simulink model "VFD.Simulink"  (R2022b)
settings: Solver=VariableStepAuto  StartTime=0.0  StopTime=5  RelTol=1e-3
libraries: spsMosfetLib x6, simulink x2, spsAsynchronousMachineSIUnitsLib x1, spsDCVoltageSourceLib x1, sps_lib x1
settings Model: Creator=Raghavendra Margam  LastModifiedBy=Raghavendra Margam

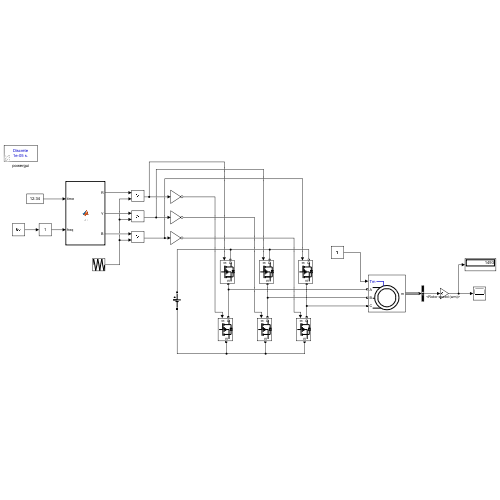
[thumbnail: Simulink's stored preview of the top-level diagram]
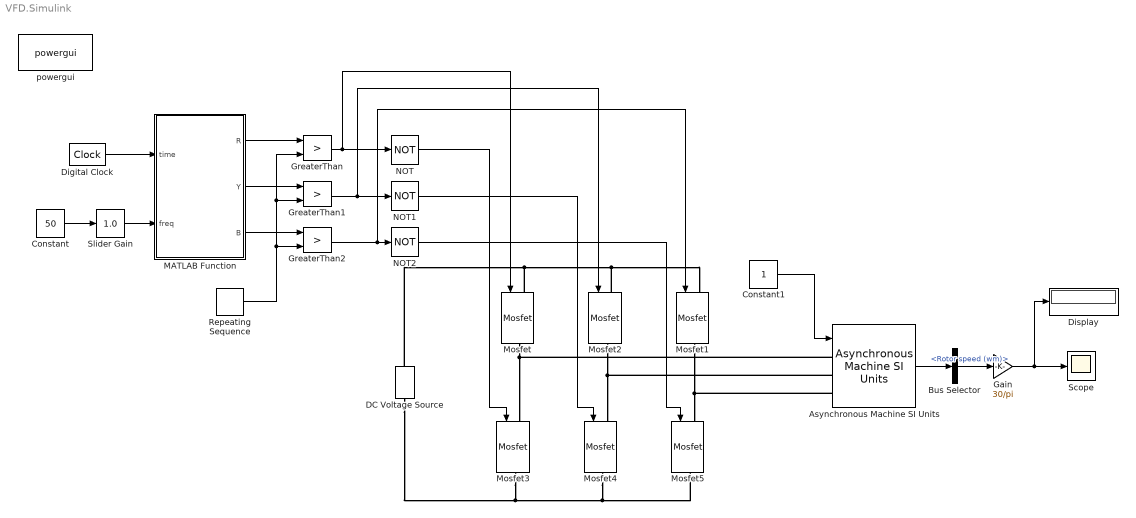
== system VFD.Simulink ==
  Asynchronous Machine SI Units : spsAsynchronousMachineSIUnitsLib/Asynchronous Machine SI Units  RotorType=Squirrel-cage  PresetModel="15:  5.4 HP (4KW)   400 V  50Hz 1430 RPM"  MechanicalLoad=Torque Tm  ShowDetailedParameters=on  ReferenceFrame=Stationary  Units=SI  MeasurementBus=off  NominalParameters=[4000 400 50]  VoltageRatio=1  Stator=[1.405 0.005839]  Rotor=[1.395 0.005839]  Cage1=[-3.163 0.003621]  Cage2=[-18.98 0.001646]  Lm=0.1722  Mechanical=[0.0131 0.002985 2]  PolePairs=2  InitialConditions=[1 0 0 0 0 0 0 0]  SimulateSaturation=off  Saturation=[14.03593122, 27.81365428, 53.79336849, 72.68890987, 97.98006896, 148.6815601, 215.7428561, 302.9841135, 428.7778367 ; 230, 322, 414, 460, 506, 552, 598, 644, 690]  LoadFlowParameters=1492000  TsPowergui=0  TsBlock=-1  IterativeModel=Trapezoidal non iterative  IterativeDiscreteModel=Trapezoidal non iterative  Pmec=1.492e+006
  Bus Selector : BusSelector  OutputSignals=Mechanical.Rotor speed (wm)
  Constant : Constant  Value=50
  Constant1 : Constant
  DC Voltage Source : spsDCVoltageSourceLib/DC Voltage Source  Amplitude=500  Measurements=None
  Digital Clock : DigitalClock  SampleTime=1e-5
  Display : Display
  Gain : Gain  Gain=30/pi
  GreaterThan : RelationalOperator  Operator=>  OutDataTypeStr=boolean  RndMeth=Simplest  InputSameDT=off
  GreaterThan1 : RelationalOperator  Operator=>  OutDataTypeStr=boolean  RndMeth=Simplest  InputSameDT=off
  GreaterThan2 : RelationalOperator  Operator=>  OutDataTypeStr=boolean  RndMeth=Simplest  InputSameDT=off
  MATLAB Function : MATLAB Function  TreatAsAtomicUnit=on
  Mosfet{,1..5} (6 alike) : spsMosfetLib/Mosfet  Ron=0.1  Lon=0  Rd=0.01  Vfd=0  IC=0  Rs=1e5  Cs=inf  Measurements=off
  NOT : Logic  Operator=NOT  IconShape=distinctive  AllPortsSameDT=off  OutDataTypeStr=boolean
  NOT1 : Logic  Operator=NOT  IconShape=distinctive  AllPortsSameDT=off  OutDataTypeStr=boolean
  NOT2 : Logic  Operator=NOT  IconShape=distinctive  AllPortsSameDT=off  OutDataTypeStr=boolean
  Repeating Sequence : simulink/Sources/Repeating Sequence  rep_seq_t=[0 .25 .5 .75 1]*1/5000  rep_seq_y=[0 1 0 -1 0]
  Scope : Scope
  Slider Gain : simulink/Math Operations/Slider Gain  gain=1.0  low=0  high=2
  powergui : sps_lib/powergui  Priority=1  SimulationMode=Discrete  SampleTime=1e-5  frequency=60  Iterations=50  frequencyindice=50  Pbase=100e6  ErrMax=1e-4  UnitsV=kV  UnitsW=MW  buscounter=0  FunctionMessages=off  echomessages=off  EnableUseOfTLC=off  CurrentSourceSwitches=off  DisableSnubberDevices=off  DisableRonSwitches=off  DisableVfSwitches=off  DisplayEquations=off  AutomaticDiscreteSolvers=off  SolverType=Tustin/Backward Euler (TBE)  Interpol=off  ExternalGateDelay=off  methode=off  Ts=100  x0status=blocks  SPID=on  SwTol=0  HookPort=off  NonlinearTolerance=1e-4  nMaxIteration=100  ContinueOnMaxIteration=off  RestoreLinks=warning  ResistiveCurrentMeasurement=off  Frange=[0:2:500]  Ylog=off  Xlog=on  ShowGrid=off  save=off  variable=ZData  structure=0  ZoomFFT=off  StartTime=0.0  cycles=1  DisplayStyle=1  fundamental=60  FreqAxis=off  MaxFrequency=1000  frequencyindicesteady=1  RmsSteady=1  display=off
  wires:
  Constant/1 -> Slider Gain/1
  Digital Clock/1 -> MATLAB Function/1(time)
  Slider Gain/1 -> MATLAB Function/2(freq)
  MATLAB Function/1(R) -> GreaterThan/1
  MATLAB Function/2(Y) -> GreaterThan1/1
  MATLAB Function/3(B) -> GreaterThan2/1
  Repeating Sequence/1 -> GreaterThan2/2, GreaterThan1/2, GreaterThan/2
  GreaterThan/1 -> NOT/1, Mosfet/1
  GreaterThan1/1 -> NOT1/1, Mosfet2/1
  GreaterThan2/1 -> Mosfet1/1, NOT2/1
  NOT/1 -> Mosfet3/1
  NOT1/1 -> Mosfet4/1
  NOT2/1 -> Mosfet5/1
  Constant1/1 -> Asynchronous Machine SI Units/1
  Asynchronous Machine SI Units/1 -> Bus Selector/1
  Bus Selector/1 -> Gain/1  "<Rotor speed (wm)>"
  Gain/1 -> Scope/1, Display/1
  connections:
  Mosfet/LConn1 -- Mosfet2/LConn1 -- Mosfet1/LConn1 -- DC Voltage Source/RConn1
  Mosfet/RConn1 -- Mosfet3/LConn1 -- Asynchronous Machine SI Units/LConn1
  Mosfet2/RConn1 -- Asynchronous Machine SI Units/LConn2 -- Mosfet4/LConn1
  Mosfet1/RConn1 -- Asynchronous Machine SI Units/LConn3 -- Mosfet5/LConn1
  Mosfet3/RConn1 -- Mosfet4/RConn1 -- Mosfet5/RConn1 -- DC Voltage Source/LConn1

== matlab function VFD.Simulink/MATLAB Function ==
  data: time input; R output; freq input; Y output; B output
function [R,Y,B] = fcn(time,freq)
omega = 2*pi*freq;
R = sin(omega*time)*freq/50;
B = sin(omega*time+120*pi/180)*freq/50;
Y = sin(omega*time+240*pi/180)*freq/50;
